simulink model "Progetto_controllore_in_s"  (Simulink 7.4)
settings: Solver=ode45  StartTime=0.0  StopTime=7  FixedStep=0.01  MaxStep=0.01  MinStep=0.0001  RelTol=1e-3
values from neighbouring files (symbols this model uses):
  den = [1 -ro*Ve*S*diam^2*Clp/(2*Ix)]    [1gdl_progetto_controllore_in_s.m]
  num = [0 ro*Ve^2*S*diam*Cldelta/Ix]    [1gdl_progetto_controllore_in_s.m]
libraries: simulink x3
settings Model: Creator=Adriano  LastModifiedBy=Adriano
settings DataIOCC: LimitDataPoints=off
settings DebuggingCC: FcnCallInpInsideContextMsg=Enable All  StrictBusMsg=ErrorLevel1

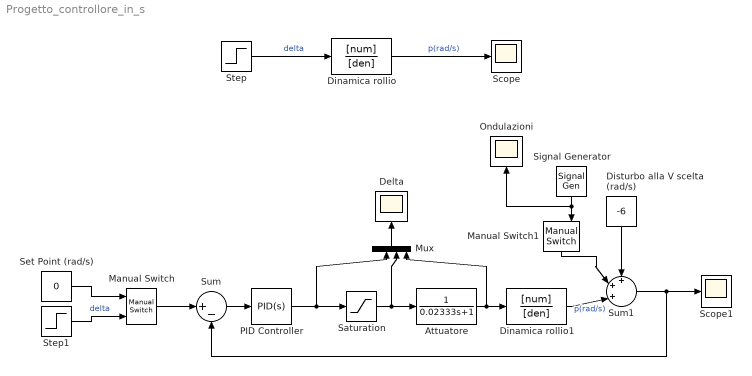
== system Progetto_controllore_in_s ==
  Attuatore : TransferFcn  Denominator=[0.02333 1]
  Delta : Scope
      settings: TimeRange=3  YMin=0  YMax=0.18  SaveName=ScopeData2
  Dinamica rollio : TransferFcn  Numerator=[num]  Denominator=[den]
  Dinamica rollio1 : TransferFcn  Numerator=[num]  Denominator=[den]
  Disturbo alla V scelta (rad/s) : Constant  Value=-6
  Manual Switch : simulink/Signal Routing/Manual Switch  SystemSampleTime=-1  sw=1  action=0  varsize=off
  Manual Switch1 : simulink/Signal Routing/Manual Switch  SystemSampleTime=-1  sw=0  action=0  varsize=off
  Mux : Mux
  Ondulazioni : Scope
      settings: TimeRange=3  YMin=0  YMax=0.18  SaveName=ScopeData3
  PID Controller : simulink/Continuous/PID Controller  DialogController=pidpack.PIDConfig.pidDDGCreate  DialogControllerArgs=DataTag0  SystemSampleTime=-1  Controller=PID  TimeDomain=Continuous-time  SampleTime=0.02  IntegratorMethod=Trapezoidal  FilterMethod=Trapezoidal  Form=Parallel  P=0.0184747470349188  I=0.8  D=1  N=0.05  InitialConditionSource=internal  InitialConditionForIntegrator=0  InitialConditionForFilter=0  ExternalReset=none  LimitOutput=on  UpperSaturationLimit=0.175  LowerSaturationLimit=-0.175  LinearizeAsGain=off  AntiWindupMode=clamping  Kb=1  TrackingMode=off  Kt=1  PParamMin=[]  PParamMax=[]  IParamMin=[]  IParamMax=[]  DParamMin=[]  DParamMax=[]  NParamMin=[]  NParamMax=[]  KbParamMin=[]  KbParamMax=[]  KtParamMin=[]  KtParamMax=[]  POutMin=[]  POutMax=[]  IOutMin=[]  IOutMax=[]  DOutMin=[]  DOutMax=[]  NOutMin=[]  NOutMax=[]  KbOutMin=[]  KbOutMax=[]  KtOutMin=[]  KtOutMax=[]  IntegratorOutMin=[]  IntegratorOutMax=[]  FilterOutMin=[]  FilterOutMax=[]  SumOutMin=[]  SumOutMax=[]  SumI1OutMin=[]  SumI1OutMax=[]  SumI2OutMin=[]  SumI2OutMax=[]  SumI3OutMin=[]  SumI3OutMax=[]  SumDOutMin=[]  SumDOutMax=[]  SaturationOutMin=[]  SaturationOutMax=[]  SaturationOutDataTypeStr=Inherit: Inherit via back propagation  IntegratorContinuousStateAttributes=''  IntegratorStateMustResolveToSignalObject=off  IntegratorRTWStateStorageClass=Auto  FilterContinuousStateAttributes=''  FilterStateMustResolveToSignalObject=off  FilterRTWStateStorageClass=Auto
  Saturation : Saturate  UpperLimit=0.175  LowerLimit=-0.175
  Scope : Scope
  Scope1 : Scope
  Set Point (rad/s) : Constant  Value=0
  Signal Generator : SignalGenerator  WaveForm=random  Amplitude=0.1  Frequency=2
  Step : Step  Time=0  After=0.174  SampleTime=0
  Step1 : Step  Before=-7  After=0  SampleTime=0
  Sum : Sum  Inputs=|+-
  Sum1 : Sum  Inputs=+++|
  wires:
  Dinamica rollio/1 -> Scope/1  "p(rad/s)"
  Step/1 -> Dinamica rollio/1  "delta"
  Sum/1 -> PID Controller/1
  PID Controller/1 -> Saturation/1, Mux/2
  Mux/1 -> Delta/1
  Sum1/1 -> Scope1/1, Sum/2
  Disturbo alla V scelta (rad/s)/1 -> Sum1/1
  Manual Switch/1 -> Sum/1
  Step1/1 -> Manual Switch/2  "delta"
  Set Point (rad/s)/1 -> Manual Switch/1
  Attuatore/1 -> Dinamica rollio1/1, Mux/4
  Saturation/1 -> Attuatore/1, Mux/3
  Dinamica rollio1/1 -> Sum1/3  "p(rad/s)"
  Signal Generator/1 -> Manual Switch1/2, Ondulazioni/1
  Manual Switch1/1 -> Sum1/2
